simulink model "unicycle_kinematic_model"  (R2022b)
settings: Solver=VariableStepAuto  StartTime=0.0  StopTime=10.0  RelTol=1e-3
libraries: robotmobilelib x1
settings Model: Creator=christian.badolo  LastModifiedBy=christian.badolo

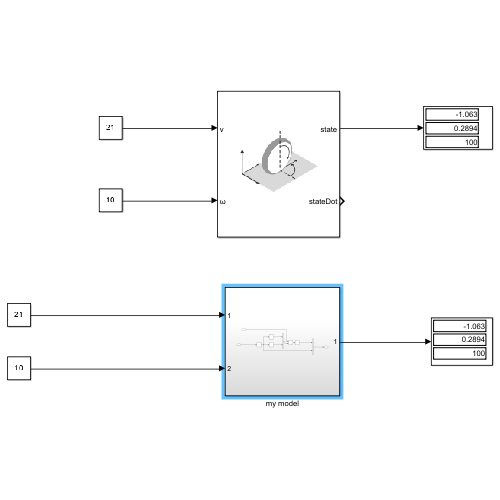
[thumbnail: Simulink's stored preview of the top-level diagram]
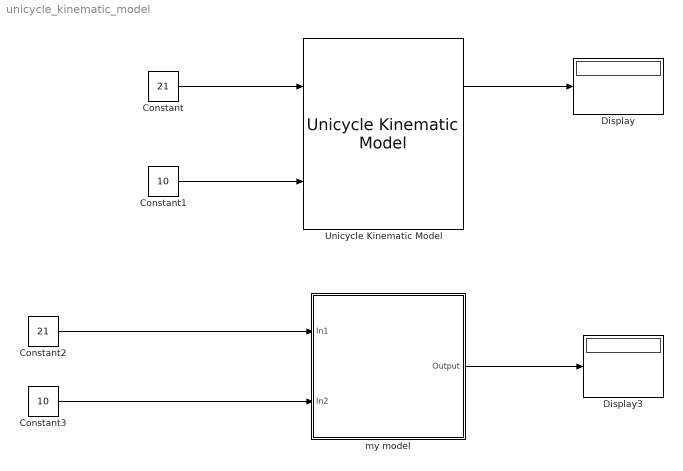
== system unicycle_kinematic_model ==
  Constant : Constant  Value=21
  Constant1 : Constant  Value=10
  Constant2 : Constant  Value=21
  Constant3 : Constant  Value=10
  Display : Display
  Display3 : Display
  Unicycle Kinematic Model : robotmobilelib/Unicycle Kinematic Model  VehicleInputs=Vehicle Speed & Heading Angular Velocity  WheelRadius=0.1  WheelSpeedRange=[-Inf Inf]  InitialState=[0; 0; 0]  SimulateUsing=Interpreted execution
  my model : Subsystem
  wires:
  Constant/1 -> Unicycle Kinematic Model/1
  Constant1/1 -> Unicycle Kinematic Model/2
  Unicycle Kinematic Model/1 -> Display/1
  my model/1(Output) -> Display3/1
  Constant2/1 -> my model/1(In1)
  Constant3/1 -> my model/2(In2)

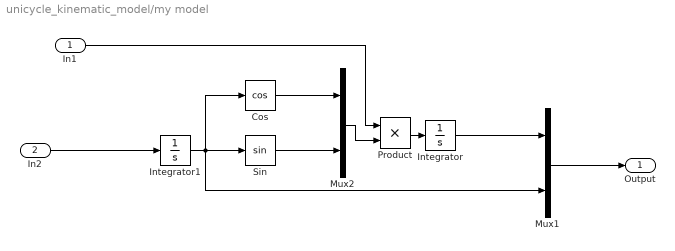
== system unicycle_kinematic_model/my model ==
  In1 : Inport
  In2 : Inport  Port=2
  Cos : Trigonometry  Operator=cos
  Integrator : Integrator
  Integrator1 : Integrator
  Mux1 : Mux  Inputs=2
  Mux2 : Mux  Inputs=2
  Product : Product
  Sin : Trigonometry
  Output : Outport
  wires:
  Integrator/1 -> Mux1/1
  Mux2/1 -> Product/2
  Product/1 -> Integrator/1
  Integrator1/1 -> Mux1/2, Sin/1, Cos/1
  In1/1 -> Product/1
  Mux1/1 -> Output/1
  Cos/1 -> Mux2/1
  Sin/1 -> Mux2/2
  In2/1 -> Integrator1/1
